simulink library "inp"  (R2021b)
settings: Solver=VariableStepAuto  StartTime=0.0  StopTime=10.0  RelTol=1e-3
undefined symbols (not defined in the file): C_TASK_5MS_S, FALSE, KINP_AcoreReadyToSlp_flg_ovrdflg, KINP_AcoreReadyToSlp_flg_ovrdval, KINP_AllowMovThd_OTA_enum_ovrdflg, KINP_AllowMovThd_OTA_enum_ovrdval, KINP_APSAngleTarget_Deg_ovrdflg, KINP_APSAngleTarget_Deg_ovrdval, KINP_APSDecReq_mps2_ovrdflg, KINP_APSDecReq_mps2_ovrdval, KINP_APSDecReqA_flg_ovrdflg, KINP_APSDecReqA_flg_ovrdval, KINP_APSDFLL_cm_ovrdflg, KINP_APSDFLL_cm_ovrdval, KINP_APSDFLR_cm_ovrdflg, KINP_APSDFLR_cm_ovrdval, KINP_APSDRLL_cm_ovrdflg, KINP_APSDRLL_cm_ovrdval, KINP_APSDRLR_cm_ovrdflg, KINP_APSDRLR_cm_ovrdval, KINP_APSExitCondition_enum_ovrdflg, KINP_APSExitCondition_enum_ovrdval, KINP_APSHWVer_enum_ovrdflg, KINP_APSHWVer_enum_ovrdval, KINP_APSProgressPCT_pct_ovrdflg, KINP_APSProgressPCT_pct_ovrdval, KINP_APSReq_enum_ovrdflg, KINP_APSReq_enum_ovrdval, KINP_APSRQDisplay_enum_ovrdflg, KINP_APSRQDisplay_enum_ovrdval, KINP_APSRqEPASCtrl_flg_ovrdflg, KINP_APSRqEPASCtrl_flg_ovrdval, KINP_APSShiftPosnReq_enum_ovrdval, KINP_APSShiftPosnReq_enum_ovrflg, KINP_APSSpeedCMD_kph_ovrdval, KINP_APSSpeedCMD_kph_ovrflg, KINP_APSStaSystem_enum_ovrdflg, KINP_APSStaSystem_enum_ovrdval, KINP_APSSWVer_enum_ovrdflg, KINP_APSSWVer_enum_ovrdval, KINP_APSVMCReqA_flg_ovrdval, KINP_APSVMCReqA_flg_ovrflg, KINP_APSVRqEPASCtrl_flg_ovrdflg, KINP_APSVRqEPASCtrl_flg_ovrdval, KINP_AuxBattVolmV_mV_ovrdflg, KINP_AuxBattVolmV_mV_ovrdval, KINP_CAASSta_enum_ovrdflg, KINP_CAASSta_enum_ovrdval, KINP_CAASVMCReqA_flg_ovrdval, KINP_CAASVMCReqA_flg_ovrflg, KINP_Chime_enum_ovrdflg, KINP_Chime_enum_ovrdval, KINP_ClearDTCcmd_flg_ovrdflg, KINP_ClearDTCcmd_flg_ovrdval, KINP_EvccAplusPwrUpReq_flg_ovrdflg, KINP_EvccAplusPwrUpReq_flg_ovrdval, KINP_LFID_raw_ovrdval, KINP_LFID_raw_ovrflg, KINP_LRID_raw_ovrdval, KINP_MemOffsetAccX_raw16_ovrdflg ... (+118)
libraries: FVT_lib x595, hcu_lib x1
(part 18 of 27)

== system inp/INP/CAN3/SignalCheck/CCU2 ==
  BHAL_outputs : Inport
  inp_CanValid_bus : Inport  Port=2
  CCU2CSErr : FVT_lib/inp/can_signal_template  SystemSampleTime=-1  VariantActivationTime=update diagram  Latency=0  AutoFrameSizeCalculation=off
      link override defval: Value=KINP_CCU2CSErr_flg_defval
      link override fftdec: Value=KINP_CCU2CSErr_flg_fftdec
      link override fftinc: Value=KINP_CCU2CSErr_flg_fftinc
      link override fftlim: Value=KINP_CCU2CSErr_flg_fftlim
      link override invalid: Value=KINP_CCU2CSErr_flg_invalid
      link override ovrdflg: Value=KINP_CCU2CSErr_flg_ovrdflg
      link override ovrdval: Value=KINP_CCU2CSErr_flg_ovrdval
      link override setvalid: Value=KINP_CCU2CSErr_flg_setvalid
      link override srvcflg: Value=KINP_CCU2CSErr_flg_srvcflg
      link override srvcval: Value=KINP_CCU2CSErr_flg_srvcval
  CCU2RCErr : FVT_lib/inp/can_signal_template  SystemSampleTime=-1  VariantActivationTime=update diagram  Latency=0  AutoFrameSizeCalculation=off
      link override defval: Value=KINP_CCU2RCErr_flg_defval
      link override fftdec: Value=KINP_CCU2RCErr_flg_fftdec
      link override fftinc: Value=KINP_CCU2RCErr_flg_fftinc
      link override fftlim: Value=KINP_CCU2RCErr_flg_fftlim
      link override invalid: Value=KINP_CCU2RCErr_flg_invalid
      link override ovrdflg: Value=KINP_CCU2RCErr_flg_ovrdflg
      link override ovrdval: Value=KINP_CCU2RCErr_flg_ovrdval
      link override setvalid: Value=KINP_CCU2RCErr_flg_setvalid
      link override srvcflg: Value=KINP_CCU2RCErr_flg_srvcflg
      link override srvcval: Value=KINP_CCU2RCErr_flg_srvcval
  CSCCU2 : FVT_lib/inp/can_signal_template  SystemSampleTime=-1  VariantActivationTime=update diagram  Latency=0  AutoFrameSizeCalculation=off
      link override defval: Value=KINP_CSCCU2_enum_defval
      link override fftdec: Value=KINP_CSCCU2_enum_fftdec
      link override fftinc: Value=KINP_CSCCU2_enum_fftinc
      link override fftlim: Value=KINP_CSCCU2_enum_fftlim
      link override invalid: Value=KINP_CSCCU2_enum_invalid
      link override ovrdflg: Value=KINP_CSCCU2_enum_ovrdflg
      link override ovrdval: Value=KINP_CSCCU2_enum_ovrdval
      link override setvalid: Value=KINP_CSCCU2_enum_setvalid
      link override srvcflg: Value=KINP_CSCCU2_enum_srvcflg
      link override srvcval: Value=KINP_CSCCU2_enum_srvcval
  DCDCEnaSta : FVT_lib/inp/can_signal_template  SystemSampleTime=-1  VariantActivationTime=update diagram  Latency=0  AutoFrameSizeCalculation=off
      link override defval: Value=KINP_DCDCEnaSta_flg_defval
      link override fftdec: Value=KINP_DCDCEnaSta_flg_fftdec
      link override fftinc: Value=KINP_DCDCEnaSta_flg_fftinc
      link override fftlim: Value=KINP_DCDCEnaSta_flg_fftlim
      link override invalid: Value=KINP_DCDCEnaSta_flg_invalid
      link override ovrdflg: Value=KINP_DCDCEnaSta_flg_ovrdflg
      link override ovrdval: Value=KINP_DCDCEnaSta_flg_ovrdval
      link override setvalid: Value=KINP_DCDCEnaSta_flg_setvalid
      link override srvcflg: Value=KINP_DCDCEnaSta_flg_srvcflg
      link override srvcval: Value=KINP_DCDCEnaSta_flg_srvcval
  DCDCFaultSta : FVT_lib/inp/can_signal_template  SystemSampleTime=-1  VariantActivationTime=update diagram  Latency=0  AutoFrameSizeCalculation=off
      link override defval: Value=KINP_DCDCFaultSta_enum_defval
      link override fftdec: Value=KINP_DCDCFaultSta_enum_fftdec
      link override fftinc: Value=KINP_DCDCFaultSta_enum_fftinc
      link override fftlim: Value=KINP_DCDCFaultSta_enum_fftlim
      link override invalid: Value=KINP_DCDCFaultSta_enum_invalid
      link override ovrdflg: Value=KINP_DCDCFaultSta_enum_ovrdflg
      link override ovrdval: Value=KINP_DCDCFaultSta_enum_ovrdval
      link override setvalid: Value=KINP_DCDCFaultSta_enum_setvalid
      link override srvcflg: Value=KINP_DCDCFaultSta_enum_srvcflg
      link override srvcval: Value=KINP_DCDCFaultSta_enum_srvcval
  DCDCReady4Pre : FVT_lib/inp/can_signal_template  SystemSampleTime=-1  VariantActivationTime=update diagram  Latency=0  AutoFrameSizeCalculation=off
      link override defval: Value=KINP_DCDCReady4Pre_flg_defval
      link override fftdec: Value=KINP_DCDCReady4Pre_flg_fftdec
      link override fftinc: Value=KINP_DCDCReady4Pre_flg_fftinc
      link override fftlim: Value=KINP_DCDCReady4Pre_flg_fftlim
      link override invalid: Value=KINP_DCDCReady4Pre_flg_invalid
      link override ovrdflg: Value=KINP_DCDCReady4Pre_flg_ovrdflg
      link override ovrdval: Value=KINP_DCDCReady4Pre_flg_ovrdval
      link override setvalid: Value=KINP_DCDCReady4Pre_flg_setvalid
      link override srvcflg: Value=KINP_DCDCReady4Pre_flg_srvcflg
      link override srvcval: Value=KINP_DCDCReady4Pre_flg_srvcval
  DCDCTemp : FVT_lib/inp/can_signal_template  SystemSampleTime=-1  VariantActivationTime=update diagram  Latency=0  AutoFrameSizeCalculation=off
      link override defval: Value=KINP_DCDCTemp_C_defval
      link override fftdec: Value=KINP_DCDCTemp_C_fftdec
      link override fftinc: Value=KINP_DCDCTemp_C_fftinc
      link override fftlim: Value=KINP_DCDCTemp_C_fftlim
      link override invalid: Value=KINP_DCDCTemp_C_invalid
      link override ovrdflg: Value=KINP_DCDCTemp_C_ovrdflg
      link override ovrdval: Value=KINP_DCDCTemp_C_ovrdval
      link override setvalid: Value=KINP_DCDCTemp_C_setvalid
      link override srvcflg: Value=KINP_DCDCTemp_C_srvcflg
      link override srvcval: Value=KINP_DCDCTemp_C_srvcval
  OBCACCurLim : FVT_lib/inp/can_signal_template  SystemSampleTime=-1  VariantActivationTime=update diagram  Latency=0  AutoFrameSizeCalculation=off
      link override defval: Value=KINP_OBCACCurLim_enum_defval
      link override fftdec: Value=KINP_OBCACCurLim_enum_fftdec
      link override fftinc: Value=KINP_OBCACCurLim_enum_fftinc
      link override fftlim: Value=KINP_OBCACCurLim_enum_fftlim
      link override invalid: Value=KINP_OBCACCurLim_enum_invalid
      link override ovrdflg: Value=KINP_OBCACCurLim_enum_ovrdflg
      link override ovrdval: Value=KINP_OBCACCurLim_enum_ovrdval
      link override setvalid: Value=KINP_OBCACCurLim_enum_setvalid
      link override srvcflg: Value=KINP_OBCACCurLim_enum_srvcflg
      link override srvcval: Value=KINP_OBCACCurLim_enum_srvcval
  OBCACCurrInf : FVT_lib/inp/can_signal_template  SystemSampleTime=-1  VariantActivationTime=update diagram  Latency=0  AutoFrameSizeCalculation=off
      link override defval: Value=KINP_OBCACCurrInf_A_defval
      link override fftdec: Value=KINP_OBCACCurrInf_A_fftdec
      link override fftinc: Value=KINP_OBCACCurrInf_A_fftinc
      link override fftlim: Value=KINP_OBCACCurrInf_A_fftlim
      link override invalid: Value=KINP_OBCACCurrInf_A_invalid
      link override ovrdflg: Value=KINP_OBCACCurrInf_A_ovrdflg
      link override ovrdval: Value=KINP_OBCACCurrInf_A_ovrdval
      link override setvalid: Value=KINP_OBCACCurrInf_A_setvalid
      link override srvcflg: Value=KINP_OBCACCurrInf_A_srvcflg
      link override srvcval: Value=KINP_OBCACCurrInf_A_srvcval
  OBCACVoltInf : FVT_lib/inp/can_signal_template  SystemSampleTime=-1  VariantActivationTime=update diagram  Latency=0  AutoFrameSizeCalculation=off
      link override defval: Value=KINP_OBCACVoltInf_V_defval
      link override fftdec: Value=KINP_OBCACVoltInf_V_fftdec
      link override fftinc: Value=KINP_OBCACVoltInf_V_fftinc
      link override fftlim: Value=KINP_OBCACVoltInf_V_fftlim
      link override invalid: Value=KINP_OBCACVoltInf_V_invalid
      link override ovrdflg: Value=KINP_OBCACVoltInf_V_ovrdflg
      link override ovrdval: Value=KINP_OBCACVoltInf_V_ovrdval
      link override setvalid: Value=KINP_OBCACVoltInf_V_setvalid
      link override srvcflg: Value=KINP_OBCACVoltInf_V_srvcflg
      link override srvcval: Value=KINP_OBCACVoltInf_V_srvcval
  OBCEnaSta : FVT_lib/inp/can_signal_template  SystemSampleTime=-1  VariantActivationTime=update diagram  Latency=0  AutoFrameSizeCalculation=off
      link override defval: Value=KINP_OBCEnaSta_flg_defval
      link override fftdec: Value=KINP_OBCEnaSta_flg_fftdec
      link override fftinc: Value=KINP_OBCEnaSta_flg_fftinc
      link override fftlim: Value=KINP_OBCEnaSta_flg_fftlim
      link override invalid: Value=KINP_OBCEnaSta_flg_invalid
      link override ovrdflg: Value=KINP_OBCEnaSta_flg_ovrdflg
      link override ovrdval: Value=KINP_OBCEnaSta_flg_ovrdval
      link override setvalid: Value=KINP_OBCEnaSta_flg_setvalid
      link override srvcflg: Value=KINP_OBCEnaSta_flg_srvcflg
      link override srvcval: Value=KINP_OBCEnaSta_flg_srvcval
  OBCFaultSta : FVT_lib/inp/can_signal_template  SystemSampleTime=-1  VariantActivationTime=update diagram  Latency=0  AutoFrameSizeCalculation=off
      link override defval: Value=KINP_OBCFaultSta_enum_defval
      link override fftdec: Value=KINP_OBCFaultSta_enum_fftdec
      link override fftinc: Value=KINP_OBCFaultSta_enum_fftinc
      link override fftlim: Value=KINP_OBCFaultSta_enum_fftlim
      link override invalid: Value=KINP_OBCFaultSta_enum_invalid
      link override ovrdflg: Value=KINP_OBCFaultSta_enum_ovrdflg
      link override ovrdval: Value=KINP_OBCFaultSta_enum_ovrdval
      link override setvalid: Value=KINP_OBCFaultSta_enum_setvalid
      link override srvcflg: Value=KINP_OBCFaultSta_enum_srvcflg
      link override srvcval: Value=KINP_OBCFaultSta_enum_srvcval
  OBCPluginSta : FVT_lib/inp/can_signal_template  SystemSampleTime=-1  VariantActivationTime=update diagram  Latency=0  AutoFrameSizeCalculation=off
      link override defval: Value=KINP_OBCPluginSta_flg_defval
      link override fftdec: Value=KINP_OBCPluginSta_flg_fftdec
      link override fftinc: Value=KINP_OBCPluginSta_flg_fftinc
      link override fftlim: Value=KINP_OBCPluginSta_flg_fftlim
      link override invalid: Value=KINP_OBCPluginSta_flg_invalid
      link override ovrdflg: Value=KINP_OBCPluginSta_flg_ovrdflg
      link override ovrdval: Value=KINP_OBCPluginSta_flg_ovrdval
      link override setvalid: Value=KINP_OBCPluginSta_flg_setvalid
      link override srvcflg: Value=KINP_OBCPluginSta_flg_srvcflg
      link override srvcval: Value=KINP_OBCPluginSta_flg_srvcval
  OBCReady4Pre : FVT_lib/inp/can_signal_template  SystemSampleTime=-1  VariantActivationTime=update diagram  Latency=0  AutoFrameSizeCalculation=off
      link override defval: Value=KINP_OBCReady4Pre_flg_defval
      link override fftdec: Value=KINP_OBCReady4Pre_flg_fftdec
      link override fftinc: Value=KINP_OBCReady4Pre_flg_fftinc
      link override fftlim: Value=KINP_OBCReady4Pre_flg_fftlim
      link override invalid: Value=KINP_OBCReady4Pre_flg_invalid
      link override ovrdflg: Value=KINP_OBCReady4Pre_flg_ovrdflg
      link override ovrdval: Value=KINP_OBCReady4Pre_flg_ovrdval
      link override setvalid: Value=KINP_OBCReady4Pre_flg_setvalid
      link override srvcflg: Value=KINP_OBCReady4Pre_flg_srvcflg
      link override srvcval: Value=KINP_OBCReady4Pre_flg_srvcval
  OBCTemp : FVT_lib/inp/can_signal_template  SystemSampleTime=-1  VariantActivationTime=update diagram  Latency=0  AutoFrameSizeCalculation=off
      link override defval: Value=KINP_OBCTemp_C_defval
      link override fftdec: Value=KINP_OBCTemp_C_fftdec
      link override fftinc: Value=KINP_OBCTemp_C_fftinc
      link override fftlim: Value=KINP_OBCTemp_C_fftlim
      link override invalid: Value=KINP_OBCTemp_C_invalid
      link override ovrdflg: Value=KINP_OBCTemp_C_ovrdflg
      link override ovrdval: Value=KINP_OBCTemp_C_ovrdval
      link override setvalid: Value=KINP_OBCTemp_C_setvalid
      link override srvcflg: Value=KINP_OBCTemp_C_srvcflg
      link override srvcval: Value=KINP_OBCTemp_C_srvcval
  OBCV2LSta : FVT_lib/inp/can_signal_template  SystemSampleTime=-1  VariantActivationTime=update diagram  Latency=0  AutoFrameSizeCalculation=off
      link override defval: Value=KINP_OBCV2LSta_enum_defval
      link override fftdec: Value=KINP_OBCV2LSta_enum_fftdec
      link override fftinc: Value=KINP_OBCV2LSta_enum_fftinc
      link override fftlim: Value=KINP_OBCV2LSta_enum_fftlim
      link override invalid: Value=KINP_OBCV2LSta_enum_invalid
      link override ovrdflg: Value=KINP_OBCV2LSta_enum_ovrdflg
      link override ovrdval: Value=KINP_OBCV2LSta_enum_ovrdval
      link override setvalid: Value=KINP_OBCV2LSta_enum_setvalid
      link override srvcflg: Value=KINP_OBCV2LSta_enum_srvcflg
      link override srvcval: Value=KINP_OBCV2LSta_enum_srvcval
  RCCCU2 : FVT_lib/inp/can_signal_template  SystemSampleTime=-1  VariantActivationTime=update diagram  Latency=0  AutoFrameSizeCalculation=off
      link override defval: Value=KINP_RCCCU2_enum_defval
      link override fftdec: Value=KINP_RCCCU2_enum_fftdec
      link override fftinc: Value=KINP_RCCCU2_enum_fftinc
      link override fftlim: Value=KINP_RCCCU2_enum_fftlim
      link override invalid: Value=KINP_RCCCU2_enum_invalid
      link override ovrdflg: Value=KINP_RCCCU2_enum_ovrdflg
      link override ovrdval: Value=KINP_RCCCU2_enum_ovrdval
      link override setvalid: Value=KINP_RCCCU2_enum_setvalid
      link override srvcflg: Value=KINP_RCCCU2_enum_srvcflg
      link override srvcval: Value=KINP_RCCCU2_enum_srvcval
  Terminator_{1..17} (17 alike) : Terminator
  True_VHAL_CCU2CSErr_flg : Constant  Value=TRUE  OutDataTypeStr=boolean
  True_VHAL_CCU2RCErr_flg : Constant  Value=TRUE  OutDataTypeStr=boolean
  True_VHAL_CSCCU2_enum : Constant  Value=TRUE  OutDataTypeStr=boolean
  True_VHAL_DCDCEnaSta_flg : Constant  Value=TRUE  OutDataTypeStr=boolean
  True_VHAL_DCDCFaultSta_enum : Constant  Value=TRUE  OutDataTypeStr=boolean
  True_VHAL_DCDCReady4Pre_flg : Constant  Value=TRUE  OutDataTypeStr=boolean
  True_VHAL_DCDCTemp_C : Constant  Value=TRUE  OutDataTypeStr=boolean
  True_VHAL_OBCACCurLim_enum : Constant  Value=TRUE  OutDataTypeStr=boolean
  True_VHAL_OBCACCurrInf_A : Constant  Value=TRUE  OutDataTypeStr=boolean
  True_VHAL_OBCACVoltInf_V : Constant  Value=TRUE  OutDataTypeStr=boolean
  True_VHAL_OBCEnaSta_flg : Constant  Value=TRUE  OutDataTypeStr=boolean
  True_VHAL_OBCFaultSta_enum : Constant  Value=TRUE  OutDataTypeStr=boolean
  True_VHAL_OBCPluginSta_flg : Constant  Value=TRUE  OutDataTypeStr=boolean
  True_VHAL_OBCReady4Pre_flg : Constant  Value=TRUE  OutDataTypeStr=boolean
  True_VHAL_OBCTemp_C : Constant  Value=TRUE  OutDataTypeStr=boolean
  True_VHAL_OBCV2LSta_enum : Constant  Value=TRUE  OutDataTypeStr=boolean
  True_VHAL_RCCCU2_enum : Constant  Value=TRUE  OutDataTypeStr=boolean
  slr1_{1..17} (17 alike) : BusSelector  OutputSignals=VINP_CANMsgValidCCU2_flg
  slr_VHAL_CCU2CSErr_flg : BusSelector  OutputSignals=VHAL_CCU2CSErr_flg
  slr_VHAL_CCU2RCErr_flg : BusSelector  OutputSignals=VHAL_CCU2RCErr_flg
  slr_VHAL_CSCCU2_enum : BusSelector  OutputSignals=VHAL_CSCCU2_enum
  slr_VHAL_DCDCEnaSta_flg : BusSelector  OutputSignals=VHAL_DCDCEnaSta_flg
  slr_VHAL_DCDCFaultSta_enum : BusSelector  OutputSignals=VHAL_DCDCFaultSta_enum
  slr_VHAL_DCDCReady4Pre_flg : BusSelector  OutputSignals=VHAL_DCDCReady4Pre_flg
  slr_VHAL_DCDCTemp_C : BusSelector  OutputSignals=VHAL_DCDCTemp_C
  slr_VHAL_OBCACCurLim_enum : BusSelector  OutputSignals=VHAL_OBCACCurLim_enum
  slr_VHAL_OBCACCurrInf_A : BusSelector  OutputSignals=VHAL_OBCACCurrInf_A
  slr_VHAL_OBCACVoltInf_V : BusSelector  OutputSignals=VHAL_OBCACVoltInf_V
  slr_VHAL_OBCEnaSta_flg : BusSelector  OutputSignals=VHAL_OBCEnaSta_flg
  slr_VHAL_OBCFaultSta_enum : BusSelector  OutputSignals=VHAL_OBCFaultSta_enum
  slr_VHAL_OBCPluginSta_flg : BusSelector  OutputSignals=VHAL_OBCPluginSta_flg
  slr_VHAL_OBCReady4Pre_flg : BusSelector  OutputSignals=VHAL_OBCReady4Pre_flg
  slr_VHAL_OBCTemp_C : BusSelector  OutputSignals=VHAL_OBCTemp_C
  slr_VHAL_OBCV2LSta_enum : BusSelector  OutputSignals=VHAL_OBCV2LSta_enum
  slr_VHAL_RCCCU2_enum : BusSelector  OutputSignals=VHAL_RCCCU2_enum
  VINP_CCU2CSErr_flg : Outport
  VINP_CCU2RCErr_flg : Outport  Port=2
  VINP_CSCCU2_enum : Outport  Port=3
  VINP_DCDCEnaSta_flg : Outport  Port=4
  VINP_DCDCFaultSta_enum : Outport  Port=5
  VINP_DCDCReady4Pre_flg : Outport  Port=6
  VINP_DCDCTemp_C : Outport  Port=7
  VINP_OBCACCurrInf_A : Outport  Port=8
  VINP_OBCACVoltInf_V : Outport  Port=9
  VINP_OBCEnaSta_flg : Outport  Port=10
  VINP_OBCFaultSta_enum : Outport  Port=11
  VINP_OBCPluginSta_flg : Outport  Port=12
  VINP_OBCReady4Pre_flg : Outport  Port=13
  VINP_OBCTemp_C : Outport  Port=14
  VINP_OBCV2LSta_enum : Outport  Port=15
  VINP_OBCACCurLim_enum : Outport  Port=16
  VINP_RCCCU2_enum : Outport  Port=17
  wires:
  BHAL_outputs/1 -> [BHAL_outputs]
  inp_CanValid_bus/1 -> [inp_CanValid_bus]
  [BHAL_outputs] -> slr_VHAL_CCU2CSErr_flg/1
  slr_VHAL_CCU2CSErr_flg/1 -> CCU2CSErr/1  "<VHAL_CCU2CSErr_flg>"
  True_VHAL_CCU2CSErr_flg/1 -> CCU2CSErr/2
  [inp_CanValid_bus] -> slr1_1/1
  slr1_1/1 -> CCU2CSErr/3  "<VINP_CANMsgValidCCU2_flg>"
  CCU2CSErr/1 -> VINP_CCU2CSErr_flg/1  "VINP_CCU2CSErr_flg"
  CCU2CSErr/2 -> Terminator_1/1
  [BHAL_outputs] -> slr_VHAL_CCU2RCErr_flg/1
  slr_VHAL_CCU2RCErr_flg/1 -> CCU2RCErr/1  "<VHAL_CCU2RCErr_flg>"
  True_VHAL_CCU2RCErr_flg/1 -> CCU2RCErr/2
  [inp_CanValid_bus] -> slr1_2/1
  slr1_2/1 -> CCU2RCErr/3  "<VINP_CANMsgValidCCU2_flg>"
  CCU2RCErr/1 -> VINP_CCU2RCErr_flg/1  "VINP_CCU2RCErr_flg"
  CCU2RCErr/2 -> Terminator_2/1
  [BHAL_outputs] -> slr_VHAL_CSCCU2_enum/1
  slr_VHAL_CSCCU2_enum/1 -> CSCCU2/1  "<VHAL_CSCCU2_enum>"
  True_VHAL_CSCCU2_enum/1 -> CSCCU2/2
  [inp_CanValid_bus] -> slr1_3/1
  slr1_3/1 -> CSCCU2/3  "<VINP_CANMsgValidCCU2_flg>"
  CSCCU2/1 -> VINP_CSCCU2_enum/1  "VINP_CSCCU2_enum"
  CSCCU2/2 -> Terminator_3/1
  [BHAL_outputs] -> slr_VHAL_DCDCEnaSta_flg/1
  slr_VHAL_DCDCEnaSta_flg/1 -> DCDCEnaSta/1  "<VHAL_DCDCEnaSta_flg>"
  True_VHAL_DCDCEnaSta_flg/1 -> DCDCEnaSta/2
  [inp_CanValid_bus] -> slr1_4/1
  slr1_4/1 -> DCDCEnaSta/3  "<VINP_CANMsgValidCCU2_flg>"
  DCDCEnaSta/1 -> VINP_DCDCEnaSta_flg/1  "VINP_DCDCEnaSta_flg"
  DCDCEnaSta/2 -> Terminator_4/1
  [BHAL_outputs] -> slr_VHAL_DCDCFaultSta_enum/1
  slr_VHAL_DCDCFaultSta_enum/1 -> DCDCFaultSta/1  "<VHAL_DCDCFaultSta_enum>"
  True_VHAL_DCDCFaultSta_enum/1 -> DCDCFaultSta/2
  [inp_CanValid_bus] -> slr1_5/1
  slr1_5/1 -> DCDCFaultSta/3  "<VINP_CANMsgValidCCU2_flg>"
  DCDCFaultSta/1 -> VINP_DCDCFaultSta_enum/1  "VINP_DCDCFaultSta_enum"
  DCDCFaultSta/2 -> Terminator_5/1
  [BHAL_outputs] -> slr_VHAL_DCDCReady4Pre_flg/1
  slr_VHAL_DCDCReady4Pre_flg/1 -> DCDCReady4Pre/1  "<VHAL_DCDCReady4Pre_flg>"
  True_VHAL_DCDCReady4Pre_flg/1 -> DCDCReady4Pre/2
  [inp_CanValid_bus] -> slr1_6/1
  slr1_6/1 -> DCDCReady4Pre/3  "<VINP_CANMsgValidCCU2_flg>"
  DCDCReady4Pre/1 -> VINP_DCDCReady4Pre_flg/1  "VINP_DCDCReady4Pre_flg"
  DCDCReady4Pre/2 -> Terminator_6/1
  [BHAL_outputs] -> slr_VHAL_DCDCTemp_C/1
  slr_VHAL_DCDCTemp_C/1 -> DCDCTemp/1  "<VHAL_DCDCTemp_C>"
  True_VHAL_DCDCTemp_C/1 -> DCDCTemp/2
  [inp_CanValid_bus] -> slr1_7/1
  slr1_7/1 -> DCDCTemp/3  "<VINP_CANMsgValidCCU2_flg>"
  DCDCTemp/1 -> VINP_DCDCTemp_C/1  "VINP_DCDCTemp_C"
  DCDCTemp/2 -> Terminator_7/1
  [BHAL_outputs] -> slr_VHAL_OBCACCurrInf_A/1
  slr_VHAL_OBCACCurrInf_A/1 -> OBCACCurrInf/1  "<VHAL_OBCACCurrInf_A>"
  True_VHAL_OBCACCurrInf_A/1 -> OBCACCurrInf/2
  [inp_CanValid_bus] -> slr1_8/1
  slr1_8/1 -> OBCACCurrInf/3  "<VINP_CANMsgValidCCU2_flg>"
  OBCACCurrInf/1 -> VINP_OBCACCurrInf_A/1  "VINP_OBCACCurrInf_A"
  OBCACCurrInf/2 -> Terminator_8/1
  [BHAL_outputs] -> slr_VHAL_OBCACVoltInf_V/1
  slr_VHAL_OBCACVoltInf_V/1 -> OBCACVoltInf/1  "<VHAL_OBCACVoltInf_V>"
  True_VHAL_OBCACVoltInf_V/1 -> OBCACVoltInf/2
  [inp_CanValid_bus] -> slr1_9/1
  slr1_9/1 -> OBCACVoltInf/3  "<VINP_CANMsgValidCCU2_flg>"
  OBCACVoltInf/1 -> VINP_OBCACVoltInf_V/1  "VINP_OBCACVoltInf_V"
  OBCACVoltInf/2 -> Terminator_9/1
  [BHAL_outputs] -> slr_VHAL_OBCEnaSta_flg/1
  slr_VHAL_OBCEnaSta_flg/1 -> OBCEnaSta/1  "<VHAL_OBCEnaSta_flg>"
  True_VHAL_OBCEnaSta_flg/1 -> OBCEnaSta/2
  [inp_CanValid_bus] -> slr1_10/1
  slr1_10/1 -> OBCEnaSta/3  "<VINP_CANMsgValidCCU2_flg>"
  OBCEnaSta/1 -> VINP_OBCEnaSta_flg/1  "VINP_OBCEnaSta_flg"
  OBCEnaSta/2 -> Terminator_10/1
  [BHAL_outputs] -> slr_VHAL_OBCFaultSta_enum/1
  slr_VHAL_OBCFaultSta_enum/1 -> OBCFaultSta/1  "<VHAL_OBCFaultSta_enum>"
  True_VHAL_OBCFaultSta_enum/1 -> OBCFaultSta/2
  [inp_CanValid_bus] -> slr1_11/1
  slr1_11/1 -> OBCFaultSta/3  "<VINP_CANMsgValidCCU2_flg>"
  OBCFaultSta/1 -> VINP_OBCFaultSta_enum/1  "VINP_OBCFaultSta_enum"
  OBCFaultSta/2 -> Terminator_11/1
  [BHAL_outputs] -> slr_VHAL_OBCPluginSta_flg/1
  slr_VHAL_OBCPluginSta_flg/1 -> OBCPluginSta/1  "<VHAL_OBCPluginSta_flg>"
  True_VHAL_OBCPluginSta_flg/1 -> OBCPluginSta/2
  [inp_CanValid_bus] -> slr1_12/1
  slr1_12/1 -> OBCPluginSta/3  "<VINP_CANMsgValidCCU2_flg>"
  OBCPluginSta/1 -> VINP_OBCPluginSta_flg/1  "VINP_OBCPluginSta_flg"
  OBCPluginSta/2 -> Terminator_12/1
  [BHAL_outputs] -> slr_VHAL_OBCReady4Pre_flg/1
  slr_VHAL_OBCReady4Pre_flg/1 -> OBCReady4Pre/1  "<VHAL_OBCReady4Pre_flg>"
  True_VHAL_OBCReady4Pre_flg/1 -> OBCReady4Pre/2
  [inp_CanValid_bus] -> slr1_13/1
  slr1_13/1 -> OBCReady4Pre/3  "<VINP_CANMsgValidCCU2_flg>"
  OBCReady4Pre/1 -> VINP_OBCReady4Pre_flg/1  "VINP_OBCReady4Pre_flg"
  OBCReady4Pre/2 -> Terminator_13/1
  [BHAL_outputs] -> slr_VHAL_OBCTemp_C/1
  slr_VHAL_OBCTemp_C/1 -> OBCTemp/1  "<VHAL_OBCTemp_C>"
  True_VHAL_OBCTemp_C/1 -> OBCTemp/2
  [inp_CanValid_bus] -> slr1_14/1
  slr1_14/1 -> OBCTemp/3  "<VINP_CANMsgValidCCU2_flg>"
  OBCTemp/1 -> VINP_OBCTemp_C/1  "VINP_OBCTemp_C"
  OBCTemp/2 -> Terminator_14/1
  [BHAL_outputs] -> slr_VHAL_OBCV2LSta_enum/1
  slr_VHAL_OBCV2LSta_enum/1 -> OBCV2LSta/1  "<VHAL_OBCV2LSta_enum>"
  True_VHAL_OBCV2LSta_enum/1 -> OBCV2LSta/2
  [inp_CanValid_bus] -> slr1_15/1
  slr1_15/1 -> OBCV2LSta/3  "<VINP_CANMsgValidCCU2_flg>"
  OBCV2LSta/1 -> VINP_OBCV2LSta_enum/1  "VINP_OBCV2LSta_enum"
  OBCV2LSta/2 -> Terminator_15/1
  [BHAL_outputs] -> slr_VHAL_OBCACCurLim_enum/1
  slr_VHAL_OBCACCurLim_enum/1 -> OBCACCurLim/1  "<VHAL_OBCACCurLim_enum>"
  True_VHAL_OBCACCurLim_enum/1 -> OBCACCurLim/2
  [inp_CanValid_bus] -> slr1_16/1
  slr1_16/1 -> OBCACCurLim/3  "<VINP_CANMsgValidCCU2_flg>"
  OBCACCurLim/1 -> VINP_OBCACCurLim_enum/1  "VINP_OBCACCurLim_enum"
  OBCACCurLim/2 -> Terminator_16/1
  [BHAL_outputs] -> slr_VHAL_RCCCU2_enum/1
  slr_VHAL_RCCCU2_enum/1 -> RCCCU2/1  "<VHAL_RCCCU2_enum>"
  True_VHAL_RCCCU2_enum/1 -> RCCCU2/2
  [inp_CanValid_bus] -> slr1_17/1
  slr1_17/1 -> RCCCU2/3  "<VINP_CANMsgValidCCU2_flg>"
  RCCCU2/1 -> VINP_RCCCU2_enum/1  "VINP_RCCCU2_enum"
  RCCCU2/2 -> Terminator_17/1

== system inp/INP/CAN3/SignalCheck/CCU4 ==
  BHAL_outputs : Inport
  inp_CanValid_bus : Inport  Port=2
  DCDCAuxCur : FVT_lib/inp/can_signal_template  SystemSampleTime=-1  VariantActivationTime=update diagram  Latency=0  AutoFrameSizeCalculation=off
      link override defval: Value=KINP_DCDCAuxCur_A_defval
      link override fftdec: Value=KINP_DCDCAuxCur_A_fftdec
      link override fftinc: Value=KINP_DCDCAuxCur_A_fftinc
      link override fftlim: Value=KINP_DCDCAuxCur_A_fftlim
      link override invalid: Value=KINP_DCDCAuxCur_A_invalid
      link override ovrdflg: Value=KINP_DCDCAuxCur_A_ovrdflg
      link override ovrdval: Value=KINP_DCDCAuxCur_A_ovrdval
      link override setvalid: Value=KINP_DCDCAuxCur_A_setvalid
      link override srvcflg: Value=KINP_DCDCAuxCur_A_srvcflg
      link override srvcval: Value=KINP_DCDCAuxCur_A_srvcval
  DCDCHVCur : FVT_lib/inp/can_signal_template  SystemSampleTime=-1  VariantActivationTime=update diagram  Latency=0  AutoFrameSizeCalculation=off
      link override defval: Value=KINP_DCDCHVCur_A_defval
      link override fftdec: Value=KINP_DCDCHVCur_A_fftdec
      link override fftinc: Value=KINP_DCDCHVCur_A_fftinc
      link override fftlim: Value=KINP_DCDCHVCur_A_fftlim
      link override invalid: Value=KINP_DCDCHVCur_A_invalid
      link override ovrdflg: Value=KINP_DCDCHVCur_A_ovrdflg
      link override ovrdval: Value=KINP_DCDCHVCur_A_ovrdval
      link override setvalid: Value=KINP_DCDCHVCur_A_setvalid
      link override srvcflg: Value=KINP_DCDCHVCur_A_srvcflg
      link override srvcval: Value=KINP_DCDCHVCur_A_srvcval
  Terminator_1 : Terminator
  Terminator_2 : Terminator
  True_VHAL_DCDCAuxCur_A : Constant  Value=TRUE  OutDataTypeStr=boolean
  True_VHAL_DCDCHVCur_A : Constant  Value=TRUE  OutDataTypeStr=boolean
  slr1_1 : BusSelector  OutputSignals=VINP_CANMsgValidCCU4_flg
  slr1_2 : BusSelector  OutputSignals=VINP_CANMsgValidCCU4_flg
  slr_VHAL_DCDCAuxCur_A : BusSelector  OutputSignals=VHAL_DCDCAuxCur_A
  slr_VHAL_DCDCHVCur_A : BusSelector  OutputSignals=VHAL_DCDCHVCur_A
  VINP_DCDCAuxCur_A : Outport
  VINP_DCDCHVCur_A : Outport  Port=2
  wires:
  BHAL_outputs/1 -> [BHAL_outputs]
  inp_CanValid_bus/1 -> [inp_CanValid_bus]
  [BHAL_outputs] -> slr_VHAL_DCDCAuxCur_A/1
  slr_VHAL_DCDCAuxCur_A/1 -> DCDCAuxCur/1  "<VHAL_DCDCAuxCur_A>"
  True_VHAL_DCDCAuxCur_A/1 -> DCDCAuxCur/2
  [inp_CanValid_bus] -> slr1_1/1
  slr1_1/1 -> DCDCAuxCur/3  "<VINP_CANMsgValidCCU4_flg>"
  DCDCAuxCur/1 -> VINP_DCDCAuxCur_A/1  "VINP_DCDCAuxCur_A"
  DCDCAuxCur/2 -> Terminator_1/1
  [BHAL_outputs] -> slr_VHAL_DCDCHVCur_A/1
  slr_VHAL_DCDCHVCur_A/1 -> DCDCHVCur/1  "<VHAL_DCDCHVCur_A>"
  True_VHAL_DCDCHVCur_A/1 -> DCDCHVCur/2
  [inp_CanValid_bus] -> slr1_2/1
  slr1_2/1 -> DCDCHVCur/3  "<VINP_CANMsgValidCCU4_flg>"
  DCDCHVCur/1 -> VINP_DCDCHVCur_A/1  "VINP_DCDCHVCur_A"
  DCDCHVCur/2 -> Terminator_2/1
